simulink model "digital_loop_filter"  (Simulink 8.1)
settings: Solver=ode45  StartTime=0.0  StopTime=simtime  RelTol=1e-3
values from neighbouring files (symbols this model uses):
  A2 = 1.82742    [lf_param.m]
  A3 = 0.827764    [lf_param.m]
  B1 = 2.74759    [lf_param.m]
  B2 = 2.70322    [lf_param.m]
  shift = 0    [digital_loop_filter_run.m]
  ts_in = 1/625/1e6    (= 1.6e-09)    [digital_loop_filter_run.m]
libraries: dspsigops x1
settings Model: Creator=amr  LastModifiedBy=amr
settings DataIOCC: SignalLoggingSaveFormat=Dataset
settings OptimizationCC: ExpressionDepthLimit=128
settings DebuggingCC: FcnCallInpInsideContextMsg=EnableAllAsError
settings GRTTargetCC: CombineOutputUpdateFcns=on  GRTInterface=off

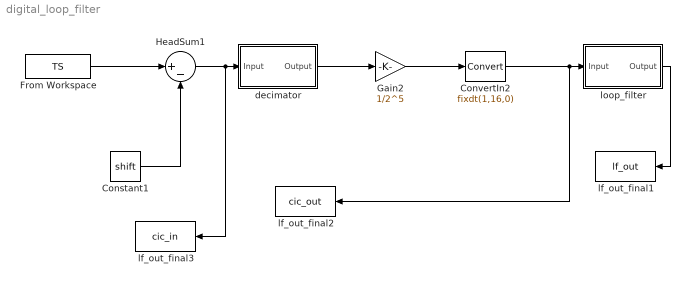
== system digital_loop_filter ==
  Constant1 : Constant  Value=shift
  ConvertIn2 : DataTypeConversion  OutDataTypeStr=fixdt(1,16,0)
  From Workspace : FromWorkspace  VariableName=TS  OutDataTypeStr=double  SampleTime=ts_in  Interpolate=off  OutputAfterFinalValue=Holding final value
  Gain2 : Gain  Gain=1/2^5  ParamDataTypeStr=double  OutDataTypeStr=double
  HeadSum1 : Sum  Inputs=|+-  AccumDataTypeStr=double  OutDataTypeStr=double  SaturateOnIntegerOverflow=on
  decimator : Subsystem  Tag=FilterWizardSubSystem
      settings: ErrorFcn=dspFilterRealizedInBasicElemsAlgLoopErrFcnCallback
  lf_out_final1 : ToWorkspace  VariableName=lf_out  SampleTime=-1
  lf_out_final2 : ToWorkspace  VariableName=cic_out  SampleTime=-1
  lf_out_final3 : ToWorkspace  VariableName=cic_in  SampleTime=-1
  loop_filter : Subsystem  Tag=FilterWizardSubSystem
      settings: ErrorFcn=dspFilterRealizedInBasicElemsAlgLoopErrFcnCallback
  wires:
  Constant1/1 -> HeadSum1/2
  From Workspace/1 -> HeadSum1/1
  HeadSum1/1 -> lf_out_final3/1, decimator/1(Input)
  decimator/1(Output) -> Gain2/1
  Gain2/1 -> ConvertIn2/1
  ConvertIn2/1 -> loop_filter/1(Input), lf_out_final2/1
  loop_filter/1(Output) -> lf_out_final1/1

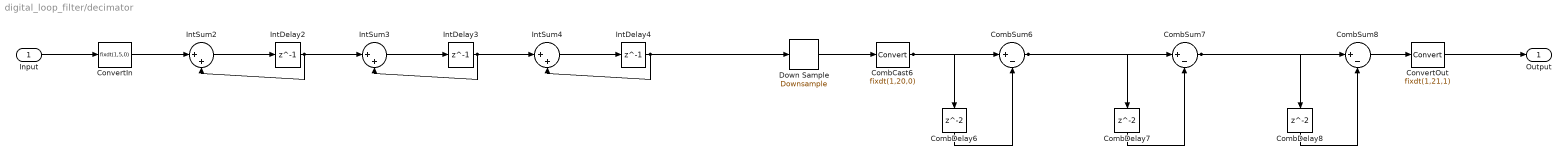
== system digital_loop_filter/decimator ==
  Input : Inport
  CombCast6 : DataTypeConversion  OutDataTypeStr=fixdt(1,20,0)
  CombDelay6 : Delay  InitialCondition=0
  CombDelay7 : Delay  InitialCondition=0
  CombDelay8 : Delay  InitialCondition=0
  CombSum6 : Sum  Inputs=|+-  AccumDataTypeStr=fixdt(1,20,0)  OutDataTypeStr=fixdt(1,20,0)
  CombSum7 : Sum  Inputs=|+-  AccumDataTypeStr=fixdt(1,20,0)  OutDataTypeStr=fixdt(1,20,0)
  CombSum8 : Sum  Inputs=|+-  AccumDataTypeStr=fixdt(1,20,0)  OutDataTypeStr=fixdt(1,20,0)
  ConvertIn : DataTypeConversion  OutDataTypeStr=fixdt(1,5,0)  RndMeth=Nearest  SaturateOnIntegerOverflow=on
  ConvertOut : DataTypeConversion  OutDataTypeStr=fixdt(1,21,1)
  Down Sample : dspsigops/Downsample  N=16  phase=0  RateOptions=Allow multirate processing  smode=Allow multirate  fmode=Maintain input frame size  ic=0
  IntDelay2 : Delay  DelayLength=1  InitialCondition=0
  IntDelay3 : Delay  DelayLength=1  InitialCondition=0
  IntDelay4 : Delay  DelayLength=1  InitialCondition=0
  IntSum2 : Sum  Inputs=|++  AccumDataTypeStr=fixdt(1,20,0)  OutDataTypeStr=fixdt(1,20,0)
  IntSum3 : Sum  Inputs=|++  AccumDataTypeStr=fixdt(1,20,0)  OutDataTypeStr=fixdt(1,20,0)
  IntSum4 : Sum  Inputs=|++  AccumDataTypeStr=fixdt(1,20,0)  OutDataTypeStr=fixdt(1,20,0)
  Output : Outport
  wires:
  Input/1 -> ConvertIn/1
  ConvertIn/1 -> IntSum2/1
  IntSum2/1 -> IntDelay2/1
  IntDelay2/1 -> IntSum2/2, IntSum3/1
  IntSum3/1 -> IntDelay3/1
  IntDelay3/1 -> IntSum3/2, IntSum4/1
  IntSum4/1 -> IntDelay4/1
  IntDelay4/1 -> IntSum4/2, Down Sample/1
  Down Sample/1 -> CombCast6/1
  CombSum6/1 -> CombSum7/1, CombDelay7/1
  CombDelay6/1 -> CombSum6/2
  CombCast6/1 -> CombSum6/1, CombDelay6/1
  CombSum7/1 -> CombSum8/1, CombDelay8/1
  CombDelay7/1 -> CombSum7/2
  CombSum8/1 -> ConvertOut/1
  CombDelay8/1 -> CombSum8/2
  ConvertOut/1 -> Output/1

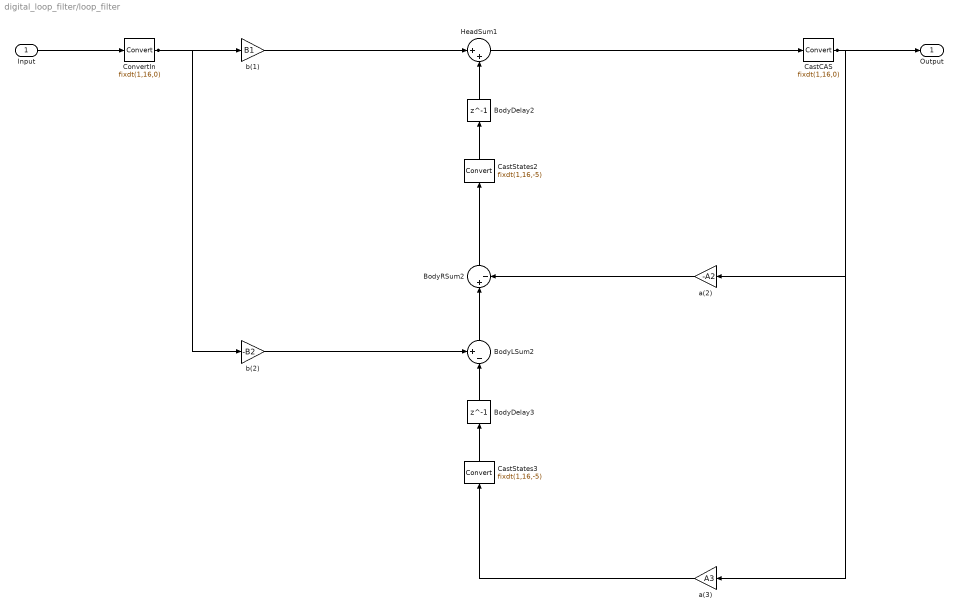
== system digital_loop_filter/loop_filter ==
  Input : Inport
  BodyDelay2 : Delay  DelayLength=1  InitialCondition=0
  BodyDelay3 : Delay  DelayLength=1  InitialCondition=0
  BodyLSum2 : Sum  Inputs=+-|  AccumDataTypeStr=fixdt(1,37,16)  OutDataTypeStr=fixdt(1,37,16)  SaturateOnIntegerOverflow=on
  BodyRSum2 : Sum  Inputs=|+-  AccumDataTypeStr=fixdt(1,37,16)  OutDataTypeStr=fixdt(1,37,16)  SaturateOnIntegerOverflow=on
  CastCAS : DataTypeConversion  OutDataTypeStr=fixdt(1,16,0)  SaturateOnIntegerOverflow=on
  CastStates2 : DataTypeConversion  OutDataTypeStr=fixdt(1,16,-5)  SaturateOnIntegerOverflow=on
  CastStates3 : DataTypeConversion  OutDataTypeStr=fixdt(1,16,-5)  SaturateOnIntegerOverflow=on
  ConvertIn : DataTypeConversion  OutDataTypeStr=fixdt(1,16,0)  RndMeth=Nearest  SaturateOnIntegerOverflow=on
  HeadSum1 : Sum  Inputs=|++  AccumDataTypeStr=fixdt(1,37,16)  OutDataTypeStr=fixdt(1,37,16)  SaturateOnIntegerOverflow=on
  a(2) : Gain  Gain=-A2  ParamDataTypeStr=fixdt(1,18,16)  OutDataTypeStr=fixdt(1,34,16)  SaturateOnIntegerOverflow=on
  a(3) : Gain  Gain=A3  ParamDataTypeStr=fixdt(1,18,16)  OutDataTypeStr=fixdt(1,34,16)  SaturateOnIntegerOverflow=on
  b(1) : Gain  Gain=B1  ParamDataTypeStr=fixdt(1,18,15)  OutDataTypeStr=fixdt(1,34,15)  SaturateOnIntegerOverflow=on
  b(2) : Gain  Gain=-B2  ParamDataTypeStr=fixdt(1,18,15)  OutDataTypeStr=fixdt(1,34,15)  SaturateOnIntegerOverflow=on
  Output : Outport
  wires:
  Input/1 -> ConvertIn/1
  b(1)/1 -> HeadSum1/1
  HeadSum1/1 -> CastCAS/1
  CastCAS/1 -> Output/1, a(2)/1, a(3)/1
  ConvertIn/1 -> b(1)/1, b(2)/1
  b(2)/1 -> BodyLSum2/1
  BodyLSum2/1 -> BodyRSum2/1
  BodyRSum2/1 -> CastStates2/1
  a(2)/1 -> BodyRSum2/2
  BodyDelay2/1 -> HeadSum1/2
  CastStates2/1 -> BodyDelay2/1
  a(3)/1 -> CastStates3/1
  BodyDelay3/1 -> BodyLSum2/2
  CastStates3/1 -> BodyDelay3/1
